simulink model "sim3"  (R2024a)
settings: Solver=FixedStepAuto  StartTime=0.0  StopTime=10.0  FixedStep=0.25  RelTol=1e-3
settings Model: Creator=alexe  LastModifiedBy=alexe

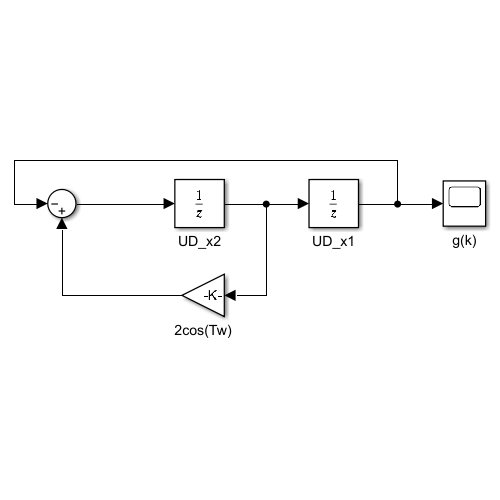
[thumbnail: Simulink's stored preview of the top-level diagram]
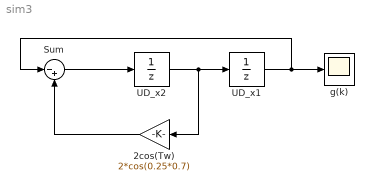
== system sim3 ==
  2cos(Tw) : Gain  Gain=2*cos(0.25*0.7)
  Sum : Sum  Inputs=|-+
  UD_x1 : UnitDelay  SampleTime=-1  HasFrameUpgradeWarning=on
  UD_x2 : UnitDelay  InitialCondition=-8.5*sin(0.25*0.7)  SampleTime=-1  HasFrameUpgradeWarning=on
  g(k) : Scope
  wires:
  UD_x2/1 -> 2cos(Tw)/1, UD_x1/1
  UD_x1/1 -> Sum/1, g(k)/1
  2cos(Tw)/1 -> Sum/2
  Sum/1 -> UD_x2/1
